simulink model "bangbang"  (Simulink 6.1)
settings: Solver=ode45  StartTime=0.0  StopTime=10.0  RelTol=1e-3
settings Model: LastModifiedBy=okawa
settings DebuggingCC: SolverPrmCheckMsg=warning

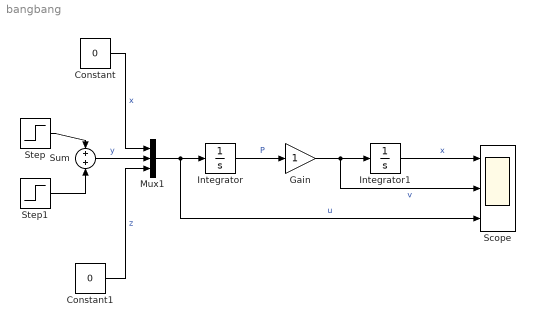
== system bangbang ==
  Constant : Constant  Value=0
  Constant1 : Constant  Value=0
  Gain : Gain
  Integrator : Integrator
  Integrator1 : Integrator
  Mux1 : Mux  Inputs=3
  Scope : Scope  NumInputPorts=3
      settings: YMin=-5~-5~-5  YMax=5~5~5
  Step : Step  SampleTime=0
  Step1 : Step  Time=2  After=-1  SampleTime=0
  Sum : Sum  Inputs=+|+
  wires:
  Constant/1 -> Mux1/1  "x"
  Constant1/1 -> Mux1/3  "z"
  Integrator1/1 -> Scope/1  "x"
  Sum/1 -> Mux1/2  "y"
  Step/1 -> Sum/1
  Step1/1 -> Sum/2
  Mux1/1 -> Integrator/1, Scope/3  "u"
  Integrator/1 -> Gain/1  "P"
  Gain/1 -> Integrator1/1, Scope/2  "v"
